simulink model "NLclose"  (R2019b)
settings: Solver=VariableStepAuto  StartTime=0.0  StopTime=50  RelTol=1e-3
values from neighbouring files (symbols this model uses):
  Ksim = SelectedController    [NLPAR.m]    (also in NOMINAL_CONTROLLER.m = Knom; RESULTS.m; WORST.m)
  NLsimpar = [segway.param.nom.m_ch   *(1 + 2*segway.param.per.delta_mch*(rand-0.5)) ... (first row only)    [NLPAR.m]
libraries: simulink x1
settings Model: Creator=Abolfazl  LastModifiedBy=Abolfazl

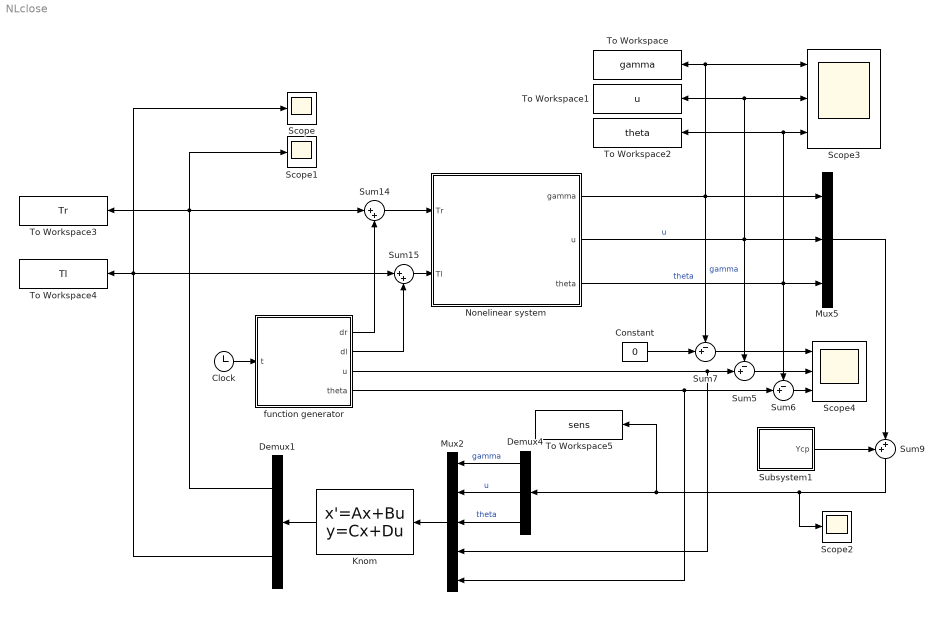
== system NLclose ==
  Clock : Clock
  Constant : Constant  Value=0
  Demux1 : Demux  Outputs=2
  Demux4 : Demux  Outputs=3
  Knom : StateSpace  A=Ksim.A  B=Ksim.B  C=Ksim.C  D=Ksim.D  InitialCondition=0
  Mux2 : Mux  Inputs=5
  Mux5 : Mux  Inputs=3
  Nonelinear system : Subsystem
  Scope : Scope
  Scope1 : Scope
  Scope2 : Scope
  Scope3 : Scope  NumInputPorts=3
  Scope4 : Scope  NumInputPorts=3
  Subsystem1 : Subsystem
  Sum14 : Sum  Inputs=|++
  Sum15 : Sum  Inputs=|++
  Sum5 : Sum  Inputs=-+|
  Sum6 : Sum  Inputs=-+|
  Sum7 : Sum  Inputs=-+|
  Sum9 : Sum  Inputs=++|
  To Workspace : ToWorkspace  VariableName=gamma  SaveFormat=Timeseries  SampleTime=-1
  To Workspace1 : ToWorkspace  VariableName=u  SaveFormat=Timeseries  SampleTime=-1
  To Workspace2 : ToWorkspace  VariableName=theta  SaveFormat=Timeseries  SampleTime=-1
  To Workspace3 : ToWorkspace  VariableName=Tr  SaveFormat=Timeseries  SampleTime=-1
  To Workspace4 : ToWorkspace  VariableName=Tl  SaveFormat=Timeseries  SampleTime=-1
  To Workspace5 : ToWorkspace  VariableName=sens  SaveFormat=Timeseries  SampleTime=-1
  function generator : MATLAB Function  TreatAsAtomicUnit=on
  wires:
  Demux4/1 -> Mux2/1  "gamma"
  function generator/4(theta) -> Mux2/5, Sum6/2
  Sum7/1 -> Scope4/1
  function generator/3(u) -> Mux2/4, Sum5/2
  Demux4/3 -> Mux2/3  "theta"
  Mux5/1 -> Sum9/2
  Sum9/1 -> Scope2/1, To Workspace5/1, Demux4/1
  Nonelinear system/1(gamma) -> Mux5/1, Scope3/1, To Workspace/1, Sum7/1  "gamma"
  Nonelinear system/2(u) -> To Workspace1/1, Scope3/2, Mux5/2, Sum5/1  "u"
  Sum6/1 -> Scope4/3
  Sum14/1 -> Nonelinear system/1(Tr)
  Demux4/2 -> Mux2/2  "u"
  Sum5/1 -> Scope4/2
  Knom/1 -> Demux1/1
  Demux1/1 -> Scope1/1, To Workspace3/1, Sum14/1
  Nonelinear system/3(theta) -> To Workspace2/1, Scope3/3, Mux5/3, Sum6/1  "theta"
  Sum15/1 -> Nonelinear system/2(Tl)
  Mux2/1 -> Knom/1
  Constant/1 -> Sum7/2
  Demux1/2 -> Scope/1, To Workspace4/1, Sum15/1
  Clock/1 -> function generator/1(t)
  function generator/2(dl) -> Sum15/2
  function generator/1(dr) -> Sum14/2
  Subsystem1/1(Ycp) -> Sum9/1

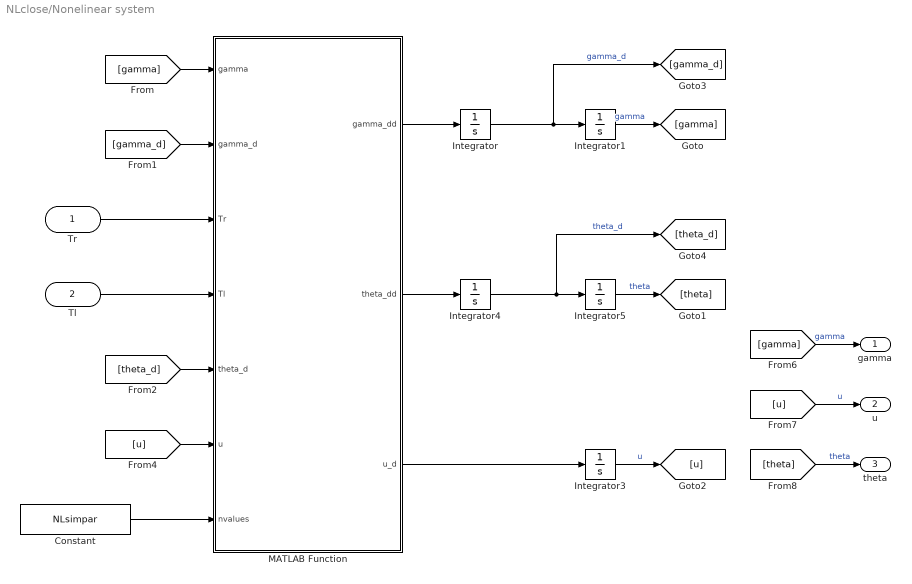
== system NLclose/Nonelinear system ==
  Tr : Inport
  Tl : Inport  Port=2
  Constant : Constant  Value=NLsimpar
  Integrator{,1,3..5} (5 alike) : Integrator
  MATLAB Function : MATLAB Function  TreatAsAtomicUnit=on
  gamma : Outport
  u : Outport  Port=2
  theta : Outport  Port=3
  wires:
  Integrator3/1 -> [u]  "u"
  MATLAB Function/1(gamma_dd) -> Integrator/1
  Integrator4/1 -> [theta_d], Integrator5/1  "theta_d"
  [gamma] -> MATLAB Function/1(gamma)
  Integrator/1 -> [gamma_d], Integrator1/1  "gamma_d"
  [theta_d] -> MATLAB Function/5(theta_d)
  [gamma_d] -> MATLAB Function/2(gamma_d)
  [theta] -> theta/1  "theta"
  [gamma] -> gamma/1  "gamma"
  [u] -> u/1  "u"
  Integrator1/1 -> [gamma]  "gamma"
  Integrator5/1 -> [theta]  "theta"
  MATLAB Function/2(theta_dd) -> Integrator4/1
  MATLAB Function/3(u_d) -> Integrator3/1
  Tr/1 -> MATLAB Function/3(Tr)
  Tl/1 -> MATLAB Function/4(Tl)
  [u] -> MATLAB Function/6(u)
  Constant/1 -> MATLAB Function/7(nvalues)

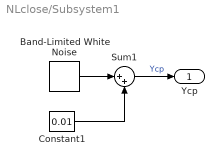
== system NLclose/Subsystem1 ==
  Band-Limited White Noise : simulink/Sources/Band-Limited White Noise  Cov=[0.001]  Ts=0.01  seed=[23341]
  Constant1 : Constant  Value=0.01
  Sum1 : Sum  Inputs=|++
  Ycp : Outport
  wires:
  Band-Limited White Noise/1 -> Sum1/1
  Constant1/1 -> Sum1/2
  Sum1/1 -> Ycp/1  "Ycp"

== matlab function NLclose/function generator ==
  settings: updateMethod=DISCRETE
  data: t input; dr output; dl output; u output; theta output
function [dr, dl, u, theta] = fcn(t)
if t>2.5
    u = 1;
else
    u = 0;
end
if t>12.5
    theta = 1;
else
    theta = 0;
end
if t>20 && t<30
    dr = 0.1;
else
    dr = 0;
end
if t>30 && t<40
    dl = 0.1;
else
    dl = 0;
end

== matlab function NLclose/Nonelinear system/MATLAB Function ==
  data: gamma input; gamma_dd output; gamma_d input; Tr input; Tl input; theta_d input; u input; theta_dd output; u_d output; nvalues input
function [gamma_dd, theta_dd, u_d] = Segway_Dynamic(gamma, gamma_d, Tr, Tl, theta_d, u, nvalues)

    m_ch   = nvalues(1);
    m_w    = nvalues(2);
    I_xx   = nvalues(3);
    I_yy   = nvalues(4); %~just in G_t
    I_zz   = nvalues(5); % Just in G_t
    I_w    = nvalues(6); % Just in G_t
    g      = nvalues(7);
    r_w    = nvalues(8);
    l      = nvalues(9);
    h      = nvalues(10);  %~Just in G_t  ------ *
    
    %--------------- Update gamma_dd --------------------------------------
    k6 = -Tl - Tr + m_ch*g*h*sin(gamma) - 0.5*(I_xx + m_ch*h^2 - I_zz)*sin(2*gamma)*theta_d^2;
    k7 = (Tr + Tl)/r_w + h*m_ch*sin(gamma)*gamma_d^2 + h*m_ch*sin(gamma)*theta_d^2 - ((3*m_w + m_ch)/(m_ch*h*cos(gamma)))*k6;
    k8 = (1/(h*m_ch*cos(gamma)))*k7;
    k9 = 1 - (3*m_w + m_ch)*(I_yy + m_ch*h^2)/((h*m_ch*cos(gamma))^2);
    gamma_dd = k8/k9;
    
    %--------------- Update theta_dd --------------------------------------
    s = (1/r_w)*Tr - (1/r_w)*Tl - m_ch*h*sin(gamma)*u*theta_d - (m_ch*h^2 + I_xx - I_zz)*sin(2*gamma)*theta_d*gamma_d;
    ss = 2*(m_w*l^2 + I_w) + I_xx*(sin(gamma)^2) + m_ch*(h^2)*(sin(gamma)^2) + I_zz*cos(gamma)^2 + m_w*l^2;
    theta_dd = s/ss;
    
    %--------------- Update u_d -------------------------------------------
    k1  = -Tr -Tl + m_ch*g*h*sin(gamma) - 0.5*(I_xx + m_ch*h^2 - I_zz)*sin(2*gamma)*theta_d^2;
    k2  = k1 - (I_yy + m_ch*h^2)*((Tr + Tl)/(h*m_ch*r_w*cos(gamma)) + tan(gamma)*(gamma_d^2 + theta_d^2));
    k3  = m_ch*h*cos(gamma) - (3*m_w + m_ch)*(I_yy + m_ch*h^2)/(h*m_ch*cos(gamma));
    u_d = k2/k3;
